simulink model "FiniteQueue_Model"  (R2024b)
settings: Solver=VariableStepAuto  StartTime=0.0  StopTime=10.0  RelTol=1e-3
libraries: NSA_DEVS_SINKS_ATOMIC x5, NSA_DEVS_LOGISTICS_ATOMIC x2, NSA_DEVS_SOURCES_ATOMIC x2, tutLib x1
settings Model: Creator=david  LastModifiedBy=peter
settings RTWCC: GPUComputeCapability=3.5

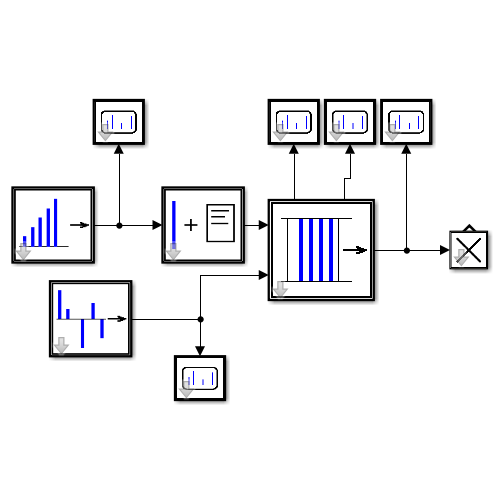
[thumbnail: Simulink's stored preview of the top-level diagram]
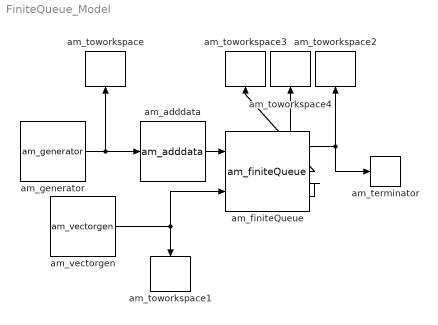
== system FiniteQueue_Model ==
  am_adddata : NSA_DEVS_LOGISTICS_ATOMIC/am_adddata  fields="[\"name\"]"  values="[\"Peter\"]"  numeric=[false]  infield="\"id\""  tau=[0,1]  debug=0
      settings: SourceProductName=Atomic
  am_finiteQueue : tutLib/am_finiteQueue  capacity=2  tD=[0,2]  tau=[0,1]  debug=0
  am_generator : NSA_DEVS_SOURCES_ATOMIC/am_generator  tG=1  n0=1  nG=100  tD=[0,2]  debug=0
      settings: SourceProductName=Atomic
  am_terminator : NSA_DEVS_LOGISTICS_ATOMIC/am_terminator  tau=[0,1]  debug=0
      settings: SourceProductName=Atomic
  am_toworkspace : NSA_DEVS_SINKS_ATOMIC/am_toworkspace  varname="\"genOut\""  t0=0  format="\"vector\""  tau=[0,1]  debug=0
      settings: SourceProductName=Atomic
  am_toworkspace1 : NSA_DEVS_SINKS_ATOMIC/am_toworkspace  varname="\"vgenOut\""  t0=0  format="\"vector\""  tau=[0,1]  debug=0
      settings: SourceProductName=Atomic
  am_toworkspace2 : NSA_DEVS_SINKS_ATOMIC/am_toworkspace  varname="\"queOut\""  t0=0  format="\"vector\""  tau=[0,1]  debug=0
      settings: SourceProductName=Atomic
  am_toworkspace3 : NSA_DEVS_SINKS_ATOMIC/am_toworkspace  varname="\"queNOut\""  t0=0  format="\"vector\""  tau=[0,1]  debug=0
      settings: SourceProductName=Atomic
  am_toworkspace4 : NSA_DEVS_SINKS_ATOMIC/am_toworkspace  varname="\"queFull\""  t0=0  format="\"vector\""  tau=[0,1]  debug=0
      settings: SourceProductName=Atomic
  am_vectorgen : NSA_DEVS_SOURCES_ATOMIC/am_vectorgen  tvec=[0.1 4.5 6.5 9.0 11.0 100]  yvec="[\"1\" \"0\" \"1\" \"0\" \"1\" \"1\"]"  tau=[0,1]  debug=0
      settings: SourceProductName=Atomic
  wires:
  am_generator/1 -> am_adddata/1, am_toworkspace/1
  am_finiteQueue/1 -> am_toworkspace2/1, am_terminator/1
  am_vectorgen/1 -> am_finiteQueue/2, am_toworkspace1/1
  am_finiteQueue/2 -> am_toworkspace3/1
  am_finiteQueue/3 -> am_toworkspace4/1
  am_adddata/1 -> am_finiteQueue/1
